simulink model "bpcheck_ver1_1"  (R2020b)
settings: Solver=VariableStepAuto  StartTime=0.0  StopTime=10.0  RelTol=1e-3
settings Model: Creator=HP  LastModifiedBy=HP

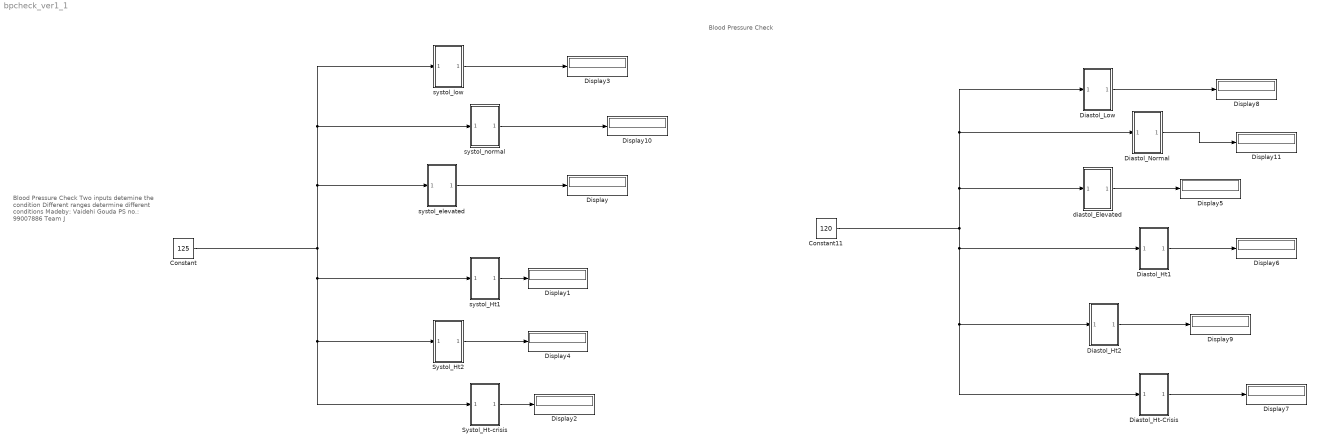
== system bpcheck_ver1_1 ==
  note: Blood Pressure Check
      |
      | Two inputs detemine the condition
      | Different ranges determine different conditions
      |
      | Madeby: Vaidehi Gouda
      | PS no.: 99007886
      | Team J
  note: Blood Pressure Check
  Constant : Constant  Value=125
  Constant11 : Constant  Value=120
  Diastol_Ht-Crisis : Subsystem
  Diastol_Ht1 : Subsystem
  Diastol_Ht2 : Subsystem
  Diastol_Low : Subsystem
  Diastol_Normal : Subsystem
  Display{,1..11} (12 alike) : Display
  Systol_Ht-crisis : Subsystem
  Systol_Ht2 : Subsystem
  diastol_Elevated : Subsystem
  systol_Ht1 : Subsystem
  systol_elevated : Subsystem
  systol_low : Subsystem
  systol_normal : Subsystem
  wires:
  Constant/1 -> Systol_Ht-crisis/1(In1), Systol_Ht2/1(In1), systol_Ht1/1(In1), systol_low/1(In1), systol_normal/1(In1), systol_elevated/1(In1)
  Constant11/1 -> Diastol_Ht-Crisis/1(In1), Diastol_Ht2/1(In1), Diastol_Ht1/1(In1), Diastol_Low/1(In1), Diastol_Normal/1(In1), diastol_Elevated/1(In1)
  systol_Ht1/1(Out1) -> Display1/1
  Systol_Ht2/1(Out1) -> Display4/1
  Systol_Ht-crisis/1(Out1) -> Display2/1
  Diastol_Low/1(Out1) -> Display8/1
  Diastol_Normal/1(Out1) -> Display11/1
  diastol_Elevated/1(Out1) -> Display5/1
  Diastol_Ht1/1(Out1) -> Display6/1
  Diastol_Ht2/1(Out1) -> Display9/1
  Diastol_Ht-Crisis/1(Out1) -> Display7/1
  systol_low/1(Out1) -> Display3/1
  systol_normal/1(Out1) -> Display10/1
  systol_elevated/1(Out1) -> Display/1

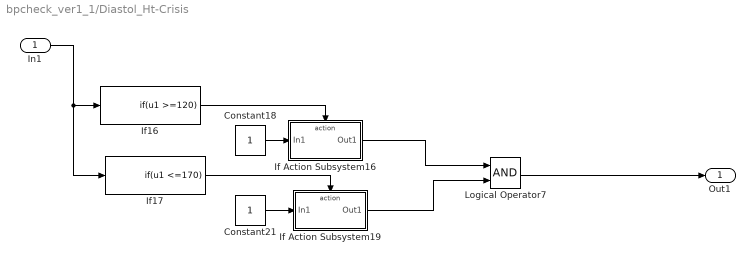
== system bpcheck_ver1_1/Diastol_Ht-Crisis ==
  In1 : Inport
  Constant18 : Constant
  Constant21 : Constant
  If Action Subsystem16 : Subsystem  TreatAsAtomicUnit=on
  If Action Subsystem19 : Subsystem  TreatAsAtomicUnit=on
  If16 : If  IfExpression=u1 >=120  ShowElse=off
  If17 : If  IfExpression=u1 <=170  ShowElse=off
  Logical Operator7 : Logic  AllPortsSameDT=off  OutDataTypeStr=boolean
  Out1 : Outport
  wires:
  If Action Subsystem19/1(Out1) -> Logical Operator7/2
  Constant18/1 -> If Action Subsystem16/1(In1)
  In1/1 -> If17/1, If16/1
  If Action Subsystem16/1(Out1) -> Logical Operator7/1
  If16/1 -> If Action Subsystem16/Action
  Constant21/1 -> If Action Subsystem19/1(In1)
  If17/1 -> If Action Subsystem19/Action
  Logical Operator7/1 -> Out1/1

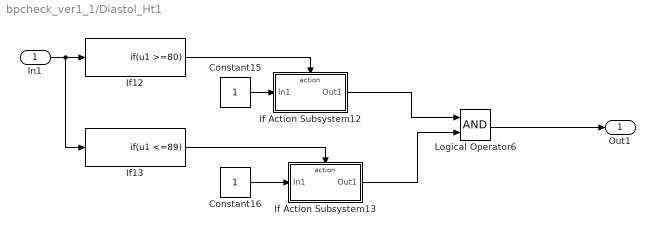
== system bpcheck_ver1_1/Diastol_Ht1 ==
  In1 : Inport
  Constant15 : Constant
  Constant16 : Constant
  If Action Subsystem12 : Subsystem  TreatAsAtomicUnit=on
  If Action Subsystem13 : Subsystem  TreatAsAtomicUnit=on
  If12 : If  IfExpression=u1 >=80  ShowElse=off
  If13 : If  IfExpression=u1 <=89  ShowElse=off
  Logical Operator6 : Logic  AllPortsSameDT=off  OutDataTypeStr=boolean
  Out1 : Outport
  wires:
  If12/1 -> If Action Subsystem12/Action
  If Action Subsystem12/1(Out1) -> Logical Operator6/1
  Constant16/1 -> If Action Subsystem13/1(In1)
  If Action Subsystem13/1(Out1) -> Logical Operator6/2
  Constant15/1 -> If Action Subsystem12/1(In1)
  In1/1 -> If13/1, If12/1
  If13/1 -> If Action Subsystem13/Action
  Logical Operator6/1 -> Out1/1

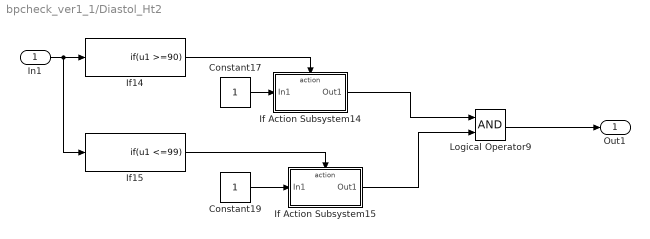
== system bpcheck_ver1_1/Diastol_Ht2 ==
  In1 : Inport
  Constant17 : Constant
  Constant19 : Constant
  If Action Subsystem14 : Subsystem  TreatAsAtomicUnit=on
  If Action Subsystem15 : Subsystem  TreatAsAtomicUnit=on
  If14 : If  IfExpression=u1 >=90  ShowElse=off
  If15 : If  IfExpression=u1 <=99  ShowElse=off
  Logical Operator9 : Logic  AllPortsSameDT=off  OutDataTypeStr=boolean
  Out1 : Outport
  wires:
  If14/1 -> If Action Subsystem14/Action
  In1/1 -> If15/1, If14/1
  Constant17/1 -> If Action Subsystem14/1(In1)
  If Action Subsystem15/1(Out1) -> Logical Operator9/2
  If15/1 -> If Action Subsystem15/Action
  Constant19/1 -> If Action Subsystem15/1(In1)
  If Action Subsystem14/1(Out1) -> Logical Operator9/1
  Logical Operator9/1 -> Out1/1

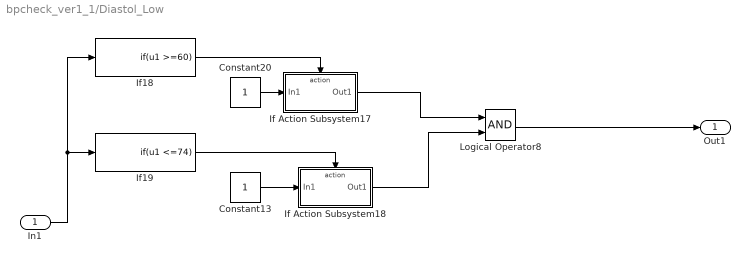
== system bpcheck_ver1_1/Diastol_Low ==
  In1 : Inport
  Constant13 : Constant
  Constant20 : Constant
  If Action Subsystem17 : Subsystem  TreatAsAtomicUnit=on
  If Action Subsystem18 : Subsystem  TreatAsAtomicUnit=on
  If18 : If  IfExpression=u1 >=60  ShowElse=off
  If19 : If  IfExpression=u1 <=74  ShowElse=off
  Logical Operator8 : Logic  AllPortsSameDT=off  OutDataTypeStr=boolean
  Out1 : Outport
  wires:
  Constant20/1 -> If Action Subsystem17/1(In1)
  If18/1 -> If Action Subsystem17/Action
  Constant13/1 -> If Action Subsystem18/1(In1)
  If Action Subsystem18/1(Out1) -> Logical Operator8/2
  If Action Subsystem17/1(Out1) -> Logical Operator8/1
  In1/1 -> If18/1, If19/1
  If19/1 -> If Action Subsystem18/Action
  Logical Operator8/1 -> Out1/1

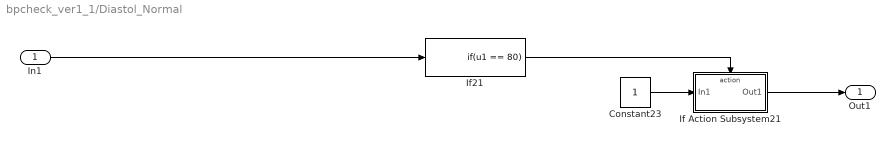
== system bpcheck_ver1_1/Diastol_Normal ==
  In1 : Inport
  Constant23 : Constant
  If Action Subsystem21 : Subsystem  TreatAsAtomicUnit=on
  If21 : If  IfExpression=u1 == 80  ShowElse=off
  Out1 : Outport
  wires:
  Constant23/1 -> If Action Subsystem21/1(In1)
  If21/1 -> If Action Subsystem21/Action
  In1/1 -> If21/1
  If Action Subsystem21/1(Out1) -> Out1/1

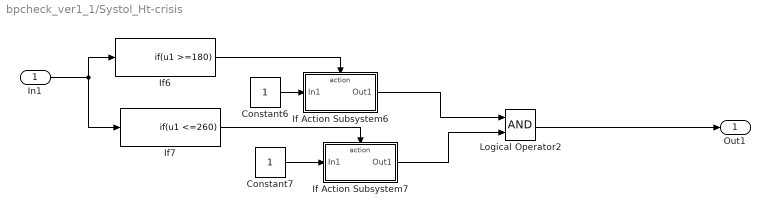
== system bpcheck_ver1_1/Systol_Ht-crisis ==
  In1 : Inport
  Constant6 : Constant
  Constant7 : Constant
  If Action Subsystem6 : Subsystem  TreatAsAtomicUnit=on
  If Action Subsystem7 : Subsystem  TreatAsAtomicUnit=on
  If6 : If  IfExpression=u1 >=180  ShowElse=off
  If7 : If  IfExpression=u1 <=260  ShowElse=off
  Logical Operator2 : Logic  AllPortsSameDT=off  OutDataTypeStr=boolean
  Out1 : Outport
  wires:
  Constant6/1 -> If Action Subsystem6/1(In1)
  In1/1 -> If6/1, If7/1
  Logical Operator2/1 -> Out1/1
  Constant7/1 -> If Action Subsystem7/1(In1)
  If7/1 -> If Action Subsystem7/Action
  If Action Subsystem6/1(Out1) -> Logical Operator2/1
  If6/1 -> If Action Subsystem6/Action
  If Action Subsystem7/1(Out1) -> Logical Operator2/2

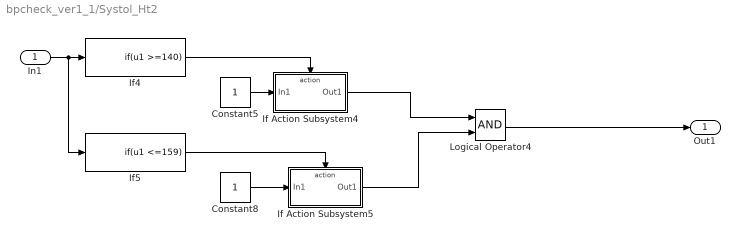
== system bpcheck_ver1_1/Systol_Ht2 ==
  In1 : Inport
  Constant5 : Constant
  Constant8 : Constant
  If Action Subsystem4 : Subsystem  TreatAsAtomicUnit=on
  If Action Subsystem5 : Subsystem  TreatAsAtomicUnit=on
  If4 : If  IfExpression=u1 >=140  ShowElse=off
  If5 : If  IfExpression=u1 <=159  ShowElse=off
  Logical Operator4 : Logic  AllPortsSameDT=off  OutDataTypeStr=boolean
  Out1 : Outport
  wires:
  Logical Operator4/1 -> Out1/1
  If5/1 -> If Action Subsystem5/Action
  If Action Subsystem4/1(Out1) -> Logical Operator4/1
  Constant8/1 -> If Action Subsystem5/1(In1)
  In1/1 -> If5/1, If4/1
  If Action Subsystem5/1(Out1) -> Logical Operator4/2
  Constant5/1 -> If Action Subsystem4/1(In1)
  If4/1 -> If Action Subsystem4/Action

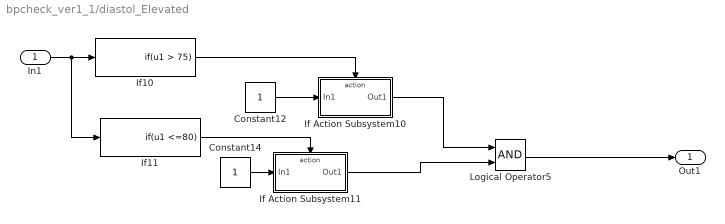
== system bpcheck_ver1_1/diastol_Elevated ==
  In1 : Inport
  Constant12 : Constant
  Constant14 : Constant
  If Action Subsystem10 : Subsystem  TreatAsAtomicUnit=on
  If Action Subsystem11 : Subsystem  TreatAsAtomicUnit=on
  If10 : If  IfExpression=u1 > 75  ShowElse=off
  If11 : If  IfExpression=u1 <=80  ShowElse=off
  Logical Operator5 : Logic  AllPortsSameDT=off  OutDataTypeStr=boolean
  Out1 : Outport
  wires:
  Constant12/1 -> If Action Subsystem10/1(In1)
  Logical Operator5/1 -> Out1/1
  If Action Subsystem11/1(Out1) -> Logical Operator5/2
  In1/1 -> If11/1, If10/1
  If Action Subsystem10/1(Out1) -> Logical Operator5/1
  Constant14/1 -> If Action Subsystem11/1(In1)
  If11/1 -> If Action Subsystem11/Action
  If10/1 -> If Action Subsystem10/Action

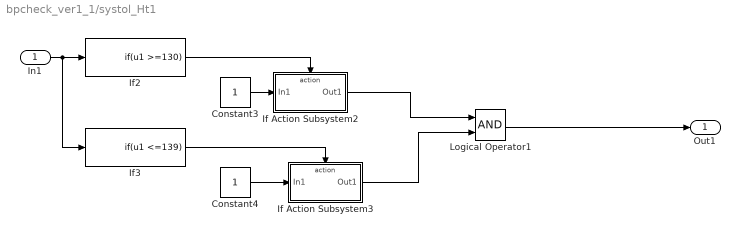
== system bpcheck_ver1_1/systol_Ht1 ==
  In1 : Inport
  Constant3 : Constant
  Constant4 : Constant
  If Action Subsystem2 : Subsystem  TreatAsAtomicUnit=on
  If Action Subsystem3 : Subsystem  TreatAsAtomicUnit=on
  If2 : If  IfExpression=u1 >=130  ShowElse=off
  If3 : If  IfExpression=u1 <=139  ShowElse=off
  Logical Operator1 : Logic  AllPortsSameDT=off  OutDataTypeStr=boolean
  Out1 : Outport
  wires:
  If2/1 -> If Action Subsystem2/Action
  Logical Operator1/1 -> Out1/1
  Constant3/1 -> If Action Subsystem2/1(In1)
  If Action Subsystem2/1(Out1) -> Logical Operator1/1
  If3/1 -> If Action Subsystem3/Action
  Constant4/1 -> If Action Subsystem3/1(In1)
  In1/1 -> If3/1, If2/1
  If Action Subsystem3/1(Out1) -> Logical Operator1/2

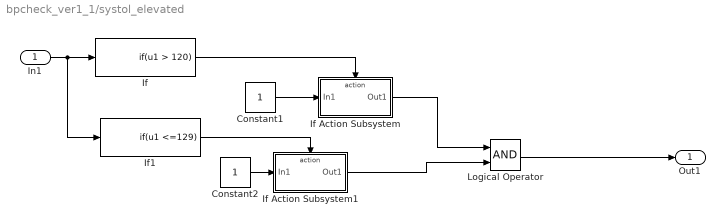
== system bpcheck_ver1_1/systol_elevated ==
  In1 : Inport
  Constant1 : Constant
  Constant2 : Constant
  If : If  IfExpression=u1 > 120  ShowElse=off
  If Action Subsystem : Subsystem  TreatAsAtomicUnit=on
  If Action Subsystem1 : Subsystem  TreatAsAtomicUnit=on
  If1 : If  IfExpression=u1 <=129  ShowElse=off
  Logical Operator : Logic  AllPortsSameDT=off  OutDataTypeStr=boolean
  Out1 : Outport
  wires:
  If Action Subsystem/1(Out1) -> Logical Operator/1
  Constant2/1 -> If Action Subsystem1/1(In1)
  If1/1 -> If Action Subsystem1/Action
  Constant1/1 -> If Action Subsystem/1(In1)
  In1/1 -> If1/1, If/1
  If/1 -> If Action Subsystem/Action
  If Action Subsystem1/1(Out1) -> Logical Operator/2
  Logical Operator/1 -> Out1/1

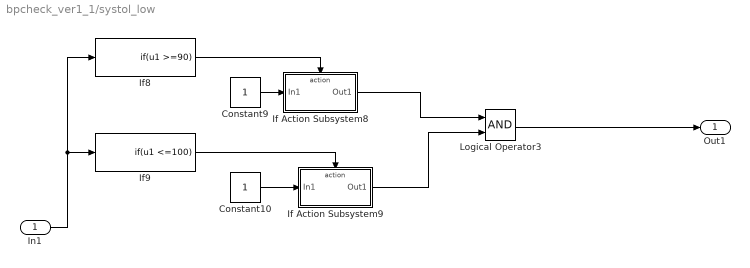
== system bpcheck_ver1_1/systol_low ==
  In1 : Inport
  Constant10 : Constant
  Constant9 : Constant
  If Action Subsystem8 : Subsystem  TreatAsAtomicUnit=on
  If Action Subsystem9 : Subsystem  TreatAsAtomicUnit=on
  If8 : If  IfExpression=u1 >=90  ShowElse=off
  If9 : If  IfExpression=u1 <=100  ShowElse=off
  Logical Operator3 : Logic  AllPortsSameDT=off  OutDataTypeStr=boolean
  Out1 : Outport
  wires:
  Constant10/1 -> If Action Subsystem9/1(In1)
  In1/1 -> If9/1, If8/1
  If Action Subsystem8/1(Out1) -> Logical Operator3/1
  If8/1 -> If Action Subsystem8/Action
  Constant9/1 -> If Action Subsystem8/1(In1)
  If9/1 -> If Action Subsystem9/Action
  If Action Subsystem9/1(Out1) -> Logical Operator3/2
  Logical Operator3/1 -> Out1/1

== system bpcheck_ver1_1/systol_normal ==
  In1 : Inport
  Constant22 : Constant
  If Action Subsystem20 : Subsystem  TreatAsAtomicUnit=on
  If20 : If  IfExpression=u1 == 120  ShowElse=off
  Out1 : Outport
  wires:
  If20/1 -> If Action Subsystem20/Action
  If Action Subsystem20/1(Out1) -> Out1/1
  Constant22/1 -> If Action Subsystem20/1(In1)
  In1/1 -> If20/1

== system bpcheck_ver1_1/Diastol_Ht-Crisis/If Action Subsystem16 ==
  In1 : Inport
  Action Port : ActionPort  ActionPortLabel=if(u1 >=120)
  Out1 : Outport
  wires:
  In1/1 -> Out1/1

== system bpcheck_ver1_1/Diastol_Ht-Crisis/If Action Subsystem19 ==
  In1 : Inport
  Action Port : ActionPort  ActionPortLabel=if(u1 <=170)
  Out1 : Outport
  wires:
  In1/1 -> Out1/1

== system bpcheck_ver1_1/Diastol_Ht1/If Action Subsystem12 ==
  In1 : Inport
  Action Port : ActionPort  ActionPortLabel=if(u1 >=80)
  Out1 : Outport
  wires:
  In1/1 -> Out1/1

== system bpcheck_ver1_1/Diastol_Ht1/If Action Subsystem13 ==
  In1 : Inport
  Action Port : ActionPort  ActionPortLabel=if(u1 <=89)
  Out1 : Outport
  wires:
  In1/1 -> Out1/1

== system bpcheck_ver1_1/Diastol_Ht2/If Action Subsystem14 ==
  In1 : Inport
  Action Port : ActionPort  ActionPortLabel=if(u1 >=90)
  Out1 : Outport
  wires:
  In1/1 -> Out1/1

== system bpcheck_ver1_1/Diastol_Ht2/If Action Subsystem15 ==
  In1 : Inport
  Action Port : ActionPort  ActionPortLabel=if(u1 <=99)
  Out1 : Outport
  wires:
  In1/1 -> Out1/1

== system bpcheck_ver1_1/Diastol_Low/If Action Subsystem17 ==
  In1 : Inport
  Action Port : ActionPort  ActionPortLabel=if(u1 >=60)
  Out1 : Outport
  wires:
  In1/1 -> Out1/1

== system bpcheck_ver1_1/Diastol_Low/If Action Subsystem18 ==
  In1 : Inport
  Action Port : ActionPort  ActionPortLabel=if(u1 <=74)
  Out1 : Outport
  wires:
  In1/1 -> Out1/1

== system bpcheck_ver1_1/Diastol_Normal/If Action Subsystem21 ==
  In1 : Inport
  Action Port : ActionPort  ActionPortLabel=if(u1 == 80)
  Out1 : Outport
  wires:
  In1/1 -> Out1/1

== system bpcheck_ver1_1/Systol_Ht-crisis/If Action Subsystem6 ==
  In1 : Inport
  Action Port : ActionPort  ActionPortLabel=if(u1 >=180)
  Out1 : Outport
  wires:
  In1/1 -> Out1/1

== system bpcheck_ver1_1/Systol_Ht-crisis/If Action Subsystem7 ==
  In1 : Inport
  Action Port : ActionPort  ActionPortLabel=if(u1 <=260)
  Out1 : Outport
  wires:
  In1/1 -> Out1/1

== system bpcheck_ver1_1/Systol_Ht2/If Action Subsystem4 ==
  In1 : Inport
  Action Port : ActionPort  ActionPortLabel=if(u1 >=140)
  Out1 : Outport
  wires:
  In1/1 -> Out1/1

== system bpcheck_ver1_1/Systol_Ht2/If Action Subsystem5 ==
  In1 : Inport
  Action Port : ActionPort  ActionPortLabel=if(u1 <=159)
  Out1 : Outport
  wires:
  In1/1 -> Out1/1

== system bpcheck_ver1_1/diastol_Elevated/If Action Subsystem10 ==
  In1 : Inport
  Action Port : ActionPort  ActionPortLabel=if(u1 > 75)
  Out1 : Outport
  wires:
  In1/1 -> Out1/1

== system bpcheck_ver1_1/diastol_Elevated/If Action Subsystem11 ==
  In1 : Inport
  Action Port : ActionPort  ActionPortLabel=if(u1 <=80)
  Out1 : Outport
  wires:
  In1/1 -> Out1/1

== system bpcheck_ver1_1/systol_Ht1/If Action Subsystem2 ==
  In1 : Inport
  Action Port : ActionPort  ActionPortLabel=if(u1 >=130)
  Out1 : Outport
  wires:
  In1/1 -> Out1/1

== system bpcheck_ver1_1/systol_Ht1/If Action Subsystem3 ==
  In1 : Inport
  Action Port : ActionPort  ActionPortLabel=if(u1 <=139)
  Out1 : Outport
  wires:
  In1/1 -> Out1/1

== system bpcheck_ver1_1/systol_elevated/If Action Subsystem ==
  In1 : Inport
  Action Port : ActionPort  ActionPortLabel=if(u1 > 120)
  Out1 : Outport
  wires:
  In1/1 -> Out1/1

== system bpcheck_ver1_1/systol_elevated/If Action Subsystem1 ==
  In1 : Inport
  Action Port : ActionPort  ActionPortLabel=if(u1 <=129)
  Out1 : Outport
  wires:
  In1/1 -> Out1/1

== system bpcheck_ver1_1/systol_low/If Action Subsystem8 ==
  In1 : Inport
  Action Port : ActionPort  ActionPortLabel=if(u1 >=90)
  Out1 : Outport
  wires:
  In1/1 -> Out1/1

== system bpcheck_ver1_1/systol_low/If Action Subsystem9 ==
  In1 : Inport
  Action Port : ActionPort  ActionPortLabel=if(u1 <=100)
  Out1 : Outport
  wires:
  In1/1 -> Out1/1

== system bpcheck_ver1_1/systol_normal/If Action Subsystem20 ==
  In1 : Inport
  Action Port : ActionPort  ActionPortLabel=if(u1 == 120)
  Out1 : Outport
  wires:
  In1/1 -> Out1/1
